simulink model "pendulum_control_final"  (R2019a)
settings: Solver=VariableStepAuto  StartTime=0.0  StopTime=10.0  RelTol=1e-3
values from neighbouring files (symbols this model uses):
  A = [0 1 0 0;(g/L) 0 0 0; 0 0 0 1; 0 0 0 0]    [inverted_pendulum.m]    (also in inverted_pendulum_final.m)
  alpha = 0.5    [inverted_pendulum_final.m]
  B = [0; (1/L); 0; 1]    [inverted_pendulum.m]    (also in inverted_pendulum_final.m = [0; -(1/L); 0; 1])
  C = [1 0 0 0; 0 0 1 0]    [inverted_pendulum.m]    (also in inverted_pendulum_final.m)
  D = [0; 0]    [inverted_pendulum.m]    (also in inverted_pendulum_final.m)
  g = 9.8    [inverted_pendulum.m]    (also in inverted_pendulum_final.m)
  ICo = 0    [inverted_pendulum_final.m]
  kbar = kpoles(2:end)    [inverted_pendulum_final.m]
  ki = kpoles(1)    [inverted_pendulum_final.m]
  L = 0.5    [inverted_pendulum.m]    (also in inverted_pendulum_final.m)
  lbar = place(A', C', pe)'    [inverted_pendulum_final.m]
settings Model: Creator=ipebo  LastModifiedBy=cgardner
settings DataIOCC: SaveFormat=Structure  ReturnWorkspaceOutputs=off
settings DebuggingCC: ArithmeticOperatorsInVariantConditions=warning

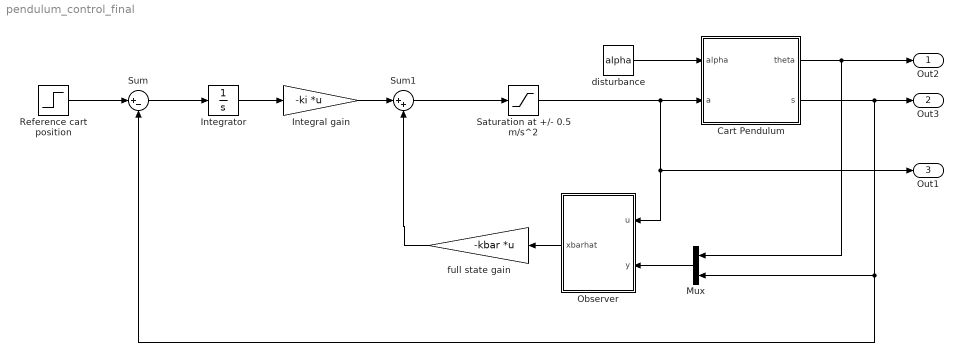
== system pendulum_control_final ==
  Cart Pendulum : Subsystem
  Integral gain : Gain  Gain=-ki  Multiplication=Matrix(K*u)
  Integrator : Integrator
  Mux : Mux  Inputs=2
  Observer : Subsystem
  Reference cart position : Step  SampleTime=0
  Saturation at +/- 0.5 m/s^2 : Saturate
  Sum : Sum  Inputs=|+-
  Sum1 : Sum  Inputs=|++
  disturbance : Constant  Value=alpha
  full state gain : Gain  Gain=-kbar  Multiplication=Matrix(K*u)
  Out2 : Outport  SignalName=theta(t)
  Out3 : Outport  Port=2  SignalName=s(t)
  Out1 : Outport  Port=3  SignalName=a(t)
  wires:
  Reference cart position/1 -> Sum/1
  Sum/1 -> Integrator/1
  Integrator/1 -> Integral gain/1
  Integral gain/1 -> Sum1/1
  Sum1/1 -> Saturation at +/- 0.5 m/s^2/1
  full state gain/1 -> Sum1/2
  Saturation at +/- 0.5 m/s^2/1 -> Cart Pendulum/2(a), Observer/1(u), Out1/1
  Observer/1(xbarhat) -> full state gain/1
  disturbance/1 -> Cart Pendulum/1(alpha)
  Cart Pendulum/1(theta) -> Mux/1, Out2/1
  Cart Pendulum/2(s) -> Out3/1, Sum/2, Mux/2
  Mux/1 -> Observer/2(y)

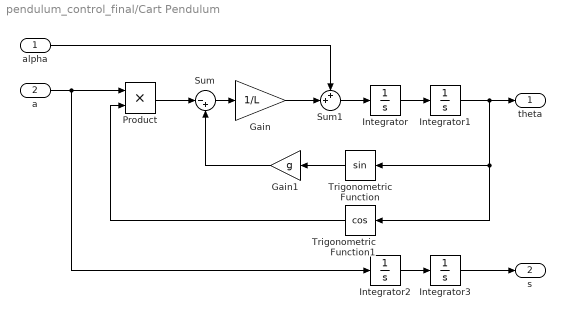
== system pendulum_control_final/Cart Pendulum ==
  alpha : Inport
  a : Inport  Port=2
  Gain : Gain  Gain=1/L
  Gain1 : Gain  Gain=g
  Integrator{,1..3} (4 alike) : Integrator
  Product : Product
  Sum : Sum  Inputs=|-+
  Sum1 : Sum  Inputs=++|
  Trigonometric Function : Trigonometry
  Trigonometric Function1 : Trigonometry  Operator=cos
  theta : Outport
  s : Outport  Port=2
  wires:
  Trigonometric Function/1 -> Gain1/1
  Integrator3/1 -> s/1
  Trigonometric Function1/1 -> Product/2
  Gain/1 -> Sum1/2
  Integrator2/1 -> Integrator3/1
  Integrator/1 -> Integrator1/1
  Product/1 -> Sum/1
  alpha/1 -> Sum1/1
  Gain1/1 -> Sum/2
  Sum1/1 -> Integrator/1
  a/1 -> Integrator2/1, Product/1
  Sum/1 -> Gain/1
  Integrator1/1 -> theta/1, Trigonometric Function1/1, Trigonometric Function/1

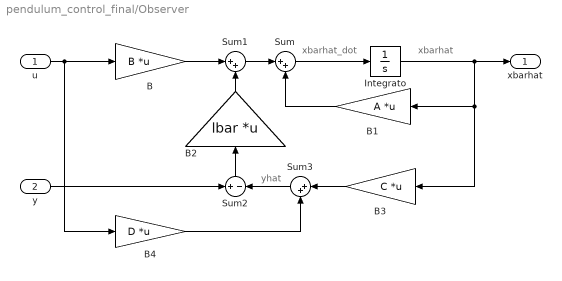
== system pendulum_control_final/Observer ==
  note: xbarhat_dot
  note: xbarhat
  note: yhat
  u : Inport
  y : Inport  Port=2
  B : Gain  Gain=B  Multiplication=Matrix(K*u)
  B1 : Gain  Gain=A  Multiplication=Matrix(K*u)
  B2 : Gain  Gain=lbar  Multiplication=Matrix(K*u)
  B3 : Gain  Gain=C  Multiplication=Matrix(K*u)
  B4 : Gain  Gain=D  Multiplication=Matrix(K*u)
  Integrato : Integrator  InitialCondition=ICo
  Sum : Sum  Inputs=|++
  Sum1 : Sum  Inputs=|++
  Sum2 : Sum  Inputs=+-
  Sum3 : Sum  Inputs=|++
  xbarhat : Outport
  wires:
  u/1 -> B/1, B4/1
  B4/1 -> Sum3/2
  y/1 -> Sum2/1
  B/1 -> Sum1/1
  Sum3/1 -> Sum2/2
  Integrato/1 -> xbarhat/1, B1/1, B3/1
  B3/1 -> Sum3/1
  Sum1/1 -> Sum/1
  B2/1 -> Sum1/2
  B1/1 -> Sum/2
  Sum/1 -> Integrato/1
  Sum2/1 -> B2/1
